simulink model "Model"  (R2014a)
settings: Solver=ode45  StartTime=0.0  StopTime=10.0  RelTol=1e-3
values from neighbouring files (symbols this model uses):
  c_phi = cos(phi)    [script.m]
  K_phi = 100    [script.m]
  s_phi = sin(phi)    [script.m]
  tau_X = 10    [script.m]
settings Model: Creator=shivjr  LastModifiedBy=shivjr

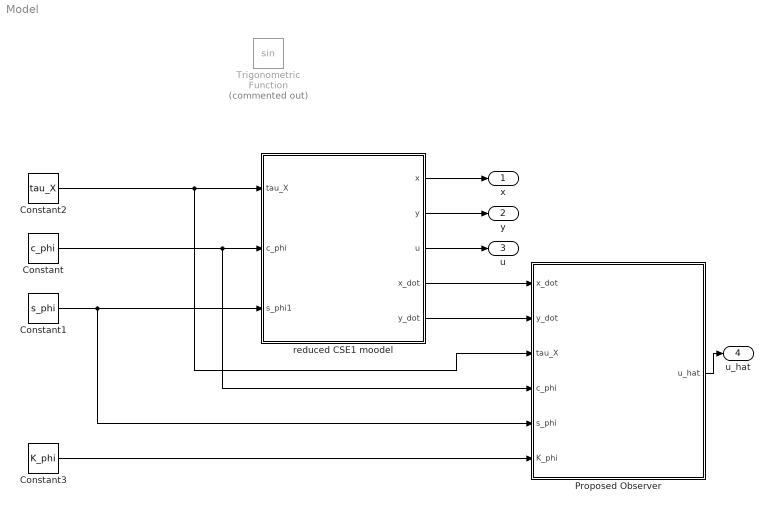
== system Model ==
  Constant : Constant  Value=c_phi
  Constant1 : Constant  Value=s_phi
  Constant2 : Constant  Value=tau_X
  Constant3 : Constant  Value=K_phi
  Proposed Observer : Subsystem
  Trigonometric Function : Trigonometry  Commented=on
  reduced CSE1 moodel : Subsystem
  x : Outport
  y : Outport  Port=2
  u : Outport  Port=3
  u_hat : Outport  Port=4
  wires:
  reduced CSE1 moodel/1(x) -> x/1
  reduced CSE1 moodel/2(y) -> y/1
  reduced CSE1 moodel/3(u) -> u/1
  Proposed Observer/1(u_hat) -> u_hat/1
  reduced CSE1 moodel/4(x_dot) -> Proposed Observer/1(x_dot)
  reduced CSE1 moodel/5(y_dot) -> Proposed Observer/2(y_dot)
  Constant/1 -> Proposed Observer/4(c_phi), reduced CSE1 moodel/2(c_phi)
  Constant1/1 -> Proposed Observer/5(s_phi), reduced CSE1 moodel/3(s_phi1)
  Constant2/1 -> Proposed Observer/3(tau_X), reduced CSE1 moodel/1(tau_X)
  Constant3/1 -> Proposed Observer/6(K_phi)

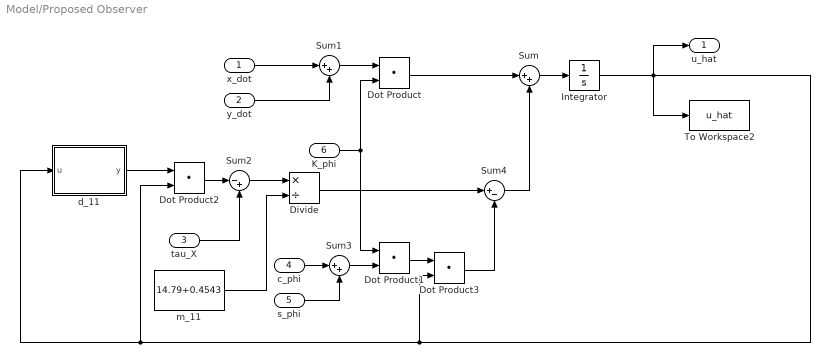
== system Model/Proposed Observer ==
  x_dot : Inport
  y_dot : Inport  Port=2
  tau_X : Inport  Port=3
  c_phi : Inport  Port=4
  s_phi : Inport  Port=5
  K_phi : Inport  Port=6
  Divide : Product  Inputs=*/
  Dot Product{,1..3} (4 alike) : DotProduct  InputSameDT=on  OutDataTypeStr=Inherit: Inherit via internal rule
  Integrator : Integrator
  Sum : Sum  Inputs=|++
  Sum1 : Sum  Inputs=|++
  Sum2 : Sum  Inputs=|-+
  Sum3 : Sum  Inputs=|++
  Sum4 : Sum  Inputs=|+-
  To Workspace2 : ToWorkspace  VariableName=u_hat  SaveFormat=Timeseries  SampleTime=-1
  d_11 : MATLAB Function  TreatAsAtomicUnit=on
  m_11 : Constant  Value=14.79+0.4543
  u_hat : Outport
  wires:
  Dot Product3/1 -> Sum4/2
  Dot Product/1 -> Sum/1
  Sum1/1 -> Dot Product/1
  x_dot/1 -> Sum1/1
  s_phi/1 -> Sum3/2
  Sum/1 -> Integrator/1
  K_phi/1 -> Dot Product/2, Dot Product1/1
  y_dot/1 -> Sum1/2
  m_11/1 -> Divide/2
  Sum2/1 -> Divide/1
  tau_X/1 -> Sum2/2
  Dot Product2/1 -> Sum2/1
  d_11/1(y) -> Dot Product2/1
  c_phi/1 -> Sum3/1
  Sum3/1 -> Dot Product1/2
  Sum4/1 -> Sum/2
  Divide/1 -> Sum4/1
  Dot Product1/1 -> Dot Product3/1
  Integrator/1 -> To Workspace2/1, u_hat/1, Dot Product3/2, Dot Product2/2, d_11/1(u)

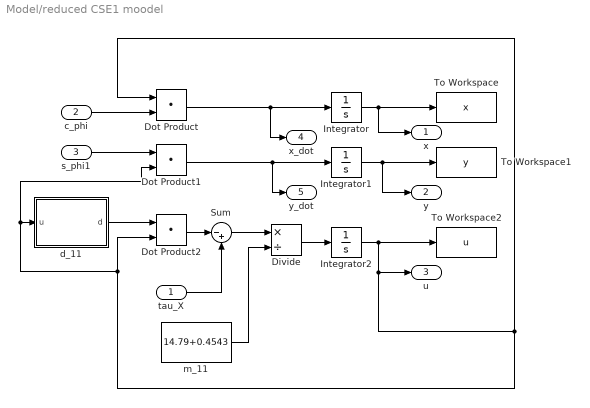
== system Model/reduced CSE1 moodel ==
  tau_X : Inport
  c_phi : Inport  Port=2
  s_phi1 : Inport  Port=3
  Divide : Product  Inputs=*/
  Dot Product : DotProduct  InputSameDT=on  OutDataTypeStr=Inherit: Inherit via internal rule
  Dot Product1 : DotProduct  InputSameDT=on  OutDataTypeStr=Inherit: Inherit via internal rule
  Dot Product2 : DotProduct  InputSameDT=on  OutDataTypeStr=Inherit: Inherit via internal rule
  Integrator : Integrator
  Integrator1 : Integrator
  Integrator2 : Integrator
  Sum : Sum  Inputs=|-+
  To Workspace : ToWorkspace  VariableName=x  SaveFormat=Timeseries  SampleTime=-1
  To Workspace1 : ToWorkspace  VariableName=y  SaveFormat=Timeseries  SampleTime=-1
  To Workspace2 : ToWorkspace  VariableName=u  SaveFormat=Timeseries  SampleTime=-1
  d_11 : MATLAB Function  TreatAsAtomicUnit=on
  m_11 : Constant  Value=14.79+0.4543
  x : Outport
  y : Outport  Port=2
  u : Outport  Port=3
  x_dot : Outport  Port=4
  y_dot : Outport  Port=5
  wires:
  Dot Product1/1 -> y_dot/1, Integrator1/1
  Integrator2/1 -> u/1, Dot Product/1, d_11/1(u), Dot Product1/2, Dot Product2/2, To Workspace2/1
  Integrator1/1 -> y/1, To Workspace1/1
  Integrator/1 -> x/1, To Workspace/1
  Dot Product/1 -> x_dot/1, Integrator/1
  d_11/1(d) -> Dot Product2/1
  Dot Product2/1 -> Sum/1
  tau_X/1 -> Sum/2
  c_phi/1 -> Dot Product/2
  s_phi1/1 -> Dot Product1/1
  Sum/1 -> Divide/1
  Divide/1 -> Integrator2/1
  m_11/1 -> Divide/2

== matlab function Model/Proposed Observer/d_11 ==
  data: u input; y output
function y = fcn(u)
%#codegen

y = u;

== matlab function Model/reduced CSE1 moodel/d_11 ==
  data: u input; d output
function d = fcn(u)
%#codegen
X_u = -0.6555;
X_uu = 0.3545;
X_uuu= -3.787;

d = -X_u - X_uu*abs(u) - X_uuu*u^2;
